simulink model "ammclib_mlib_vmac_s32k14x"  (Simulink 9.0)
settings: Solver=FixedStepDiscrete  StartTime=0.0  StopTime=5  FixedStep=0.001  RelTol=1e-3  EnableMultiTasking=on
InitFcn:
  | mbd_s32k_consistency_checks(bdroot(gcs));
undefined symbols (not defined in the file): LQFP
libraries: ammclib_bam_s32k14x x16, simulink x5, mbd_s32k1xx_ec_toolbox x2
Description:
  | This model tests the AMMCLIB MLIB VMAC blocks
  | 
  | Validation:
  | - Run the model in Simulation and compare the Inputs vs Outputs results.
  | - Open Freemaster (ammclib_mlib_vmac_s32k14x.pmp) and compare the HW results against the Simulated ones
settings Model: Creator=NXP MBDT Team  LastModifiedBy=nxf35172
settings DataIOCC: ExternalInput=off  InitialState=off  LimitDataPoints=on  SaveOutput=off  SignalLogging=off  SaveTime=off
settings OptimizationCC: DefaultParameterBehavior=Inlined  LifeSpan=1
settings DebuggingCC: SolverPrmCheckMsg=warning  InheritedTsInSrcMsg=none  SingleTaskRateTransMsg=error  ParameterPrecisionLossMsg=none  UnconnectedInputMsg=error  UnconnectedOutputMsg=error  UnconnectedLineMsg=error  AllowSymbolicDim=off  UnknownTsInhSupMsg=error  StateNameClashWarn=warning
settings HardwareCC: ProdLargestAtomicInteger=Long  ProdLargestAtomicFloat=Double  ProdEndianess=LittleEndian  ProdHWDeviceType=ARM Compatible->ARM Cortex
settings SFSimCC: MATLABDynamicMemAlloc=off
settings RTWCC: SystemTargetFile=mbd_s32k.tlc  MakeCommand=mbd_s32k_make_rtw COPY_MDLREF_INCLUDES=0  TemplateMakefile=mbd_s32k.tmf  Description=Model Based Design Toolbox S32K14x Code Generation Target
settings CodeAppCC: IgnoreCustomStorageClasses=off
settings STFCustomTargetCC: CombineOutputUpdateFcns=on  ERTCustomFileBanners=on  SupportContinuousTime=off  SupportNonInlinedSFcns=off  RemoveResetFunc=on  MATLABClassNameForMDSCustomization=Simulink.SoftwareTarget.ERTCustomization  GRTInterface=off  SystemTargetFile=mbd_s32k14.tlc
settings ERTTargetCC: MultiwordLength=2048  ParMdlRefBuildCompliant=off  CompOptLevelCompliant=off  ConcurrentExecutionCompliant=off  ModelStepFunctionPrototypeControlCompliant=off  CPPClassGenCompliant=off  UseToolchainInfoCompliant=off  InlinedParameterPlacement=NonHierarchical  ERTCustomFileTemplate=example_file_process.tlc  ConvertIfToSwitch=off  SuppressUnreachableDefaultCases=off

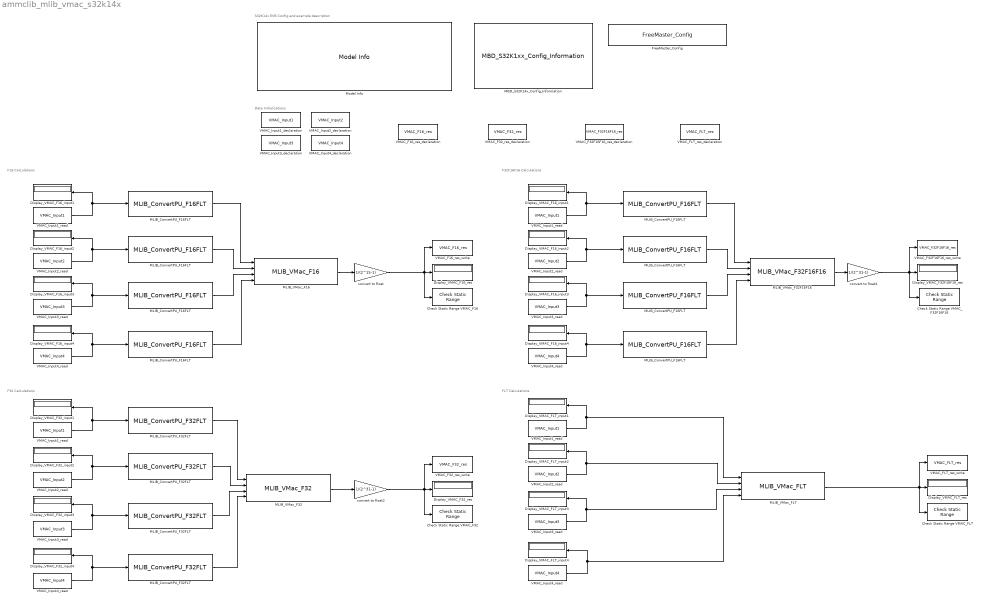
== system ammclib_mlib_vmac_s32k14x ==
  note: S32K14x EVB Config and example description
  note: Data Initializations
  note: F16 Calculations
  note: FLT Calculations
  note: F32F16F16 Calculations
  note: F32 Calculations
  "   MLIB_ConvertPU_F16FLT  " : ammclib_bam_s32k14x/MLIB/bam_f16/MLIB_ConvertPU_F16FLT
  "  MLIB_ConvertPU_F16FLT " : ammclib_bam_s32k14x/MLIB/bam_f16/MLIB_ConvertPU_F16FLT
  "  MLIB_ConvertPU_F16FLT   " : ammclib_bam_s32k14x/MLIB/bam_f16/MLIB_ConvertPU_F16FLT
  "  MLIB_ConvertPU_F16FLT     " : ammclib_bam_s32k14x/MLIB/bam_f16/MLIB_ConvertPU_F16FLT
  "  VMAC_Input4_read" : DataStoreRead  DataStoreName=VMAC_Input4
  " Display_VMAC_F16_input3" : Display
  " Display_VMAC_F16_input4" : Display
  " MLIB_ConvertPU_F16FLT" : ammclib_bam_s32k14x/MLIB/bam_f16/MLIB_ConvertPU_F16FLT
  " VMAC_Input3_read" : DataStoreRead  DataStoreName=VMAC_Input3
  Check Static Range VMAC_F16 : simulink/Model Verification/Check  Static Range  Description=0.194 <= u <= 0.196  max=0.196  max_included=on  min=0.194  min_included=on  enabled=on  stopWhenAssertionFail=on  export=off  icon=graphic
      settings: SourceProductName=Simulink  SourceProductBaseCode=SL
  "Check Static Range VMAC_F32 " : simulink/Model Verification/Check  Static Range  Description=0.194 <= u <= 0.196  max=0.196  max_included=on  min=0.194  min_included=on  enabled=on  stopWhenAssertionFail=on  export=off  icon=graphic
      settings: SourceProductName=Simulink  SourceProductBaseCode=SL
  "Check Static Range VMAC_F32F16F16 " : simulink/Model Verification/Check  Static Range  Description=0.194 <= u <= 0.196  max=0.196  max_included=on  min=0.194  min_included=on  enabled=on  stopWhenAssertionFail=on  export=off  icon=graphic
      settings: SourceProductName=Simulink  SourceProductBaseCode=SL
  "Check Static Range VMAC_FLT " : simulink/Model Verification/Check  Static Range  Description=0.194 <= u <= 0.196  max=0.196  max_included=on  min=0.194  min_included=on  enabled=on  stopWhenAssertionFail=on  export=off  icon=graphic
      settings: SourceProductName=Simulink  SourceProductBaseCode=SL
  Display_VMAC_F16_input{1..4} (4 alike) : Display
  "Display_VMAC_F16_input1   " : Display
  "Display_VMAC_F16_input2    " : Display
  Display_VMAC_F16_res : Display
  Display_VMAC_F32F16F16_res : Display
  Display_VMAC_F32_input1 : Display
  "Display_VMAC_F32_input2 " : Display
  Display_VMAC_F32_input3 : Display
  Display_VMAC_F32_input4 : Display
  Display_VMAC_F32_res : Display
  Display_VMAC_FLT_input{1..4} (4 alike) : Display
  Display_VMAC_FLT_res : Display
  FreeMaster_Config : mbd_s32k1xx_ec_toolbox/Utility Blocks/FreeMaster_Config  interface=LPUART1  baudrate=115200  rxd=PTC6: [LPUART1_RX | Receive]  txd=PTC7: [LPUART1_TX | Transmit]  mode=Short Interrupt  isr_prio=15  show_adv_opts=off  use_scope=on  max_scope_vars=8  use_recorder=on  max_rec_vars=8  rec_buff_size=1024  rec_timebase=0 milliseconds  comm_buffer_size_auto=on  comm_buffer_size=255  comm_rqueue_size_default=on  comm_rqueue_size=32
  MBD_S32K14x_Config_Information : mbd_s32k1xx_ec_toolbox/MBD_S32K1xx_Config_Information  Priority=0  mbdt_ver=0  disp_str=|  config_params=[]  mcu_target_name=S32K144  mcu_target_package=100-LQFP  mcu_target_sram_size=64KB  mcu_system_clock_freq=80  mcu_xtal_freq=External 8  mcu_steptick_timer=LPIT Channel 0  mcu_steptick_prio=15  ds_import_enable=on  target_compiler=GCC  target_memory=FLASH  gcc_target_compile_opts=-mcpu=cortex-m4 -mthumb -mfloat-abi=hard -mfpu=fpv4-sp-d16 -O1 -g -gstrict-dwarf  gcc_target_assemble_opts=-mcpu=cortex-m4 -mthumb -mfloat-abi=hard -mfpu=fpv4-sp-d16 -g  gcc_target_link_opts=-mcpu=cortex-m4 -mthumb -mfloat-abi=hard -mfpu=fpv4-sp-d16  gcc_target_default_lcf=on  gcc_target_user_lcf=S32K144_64_flash.ld  ghs_target_compile_opts=-cpu=cortexm4f -thumb -DARM_MATH_CM4 -fpu=vfpv4_d16 -fsingle -Ogeneral -Wundef -Wimplicit-int -Wshadow -Wtrigraphs --no_commons --gnu_asm -gnu99 -gdwarf-2 -G  ghs_target_assemble_opts=-cpu=cortexm4f -fpu=vfpv4_d16  ghs_target_link_opts=-cpu=cortexm4f -thumb -fpu=vfpv4_d16  ghs_target_default_lcf=off  ghs_target_user_lcf=S32K144_64_flash.ld  iar_target_compile_opts=--cpu=Cortex-M4F --thumb --fpu=VFPv4_sp -Ol -e --debug --dlib_config normal  iar_target_assemble_opts=--cpu Cortex-M4F --thumb --fpu VFPv4_sp  iar_target_link_opts=--no_exceptions --vfe --inline  iar_target_default_lcf=off  iar_target_user_lcf=S32K144_64_flash.icf  pil_download_enable=off  rbl_download_enable=on  rbl_start_delay=5000000  rbl_download_interface=OpenSDA  rbl_restart_request=off  rbl_com_port=Custom  rbl_com_port_custom=COM1  pil_download_rate=57600  pil_opensda_drive=Custom  pil_opensda_drive_custom=D  pil_uart_instance=1  pil_uart_rx=PTC6: [LPUART1_RX | Receive]  pil_uart_tx=PTC7: [LPUART1_TX | Transmit]  FTM_PWM_PcrCheckEnDis=on  FTM_Input_Edge_Inputs_PcrCheckEnDis=on  FTM_Dual_Edge_Inputs_PcrCheckEnDis=on  FTM_Quadrature_Inputs_PcrCheckEnDis=on  FTM_Hall_Sensor_Inputs_PcrCheckEnDis=on  LPTMR_PcrCheckEnDis=on  PIT_PcrCheckEnDis=on  RTC_PcrCheckEnDis=on  FlexCAN_PcrCheckEnDis=on  LIN_PcrCheckEnDis=on  FlexIO_PcrCheckEnDis=on  LPI2C_PcrCheckEnDis=on  LPSPI_PcrCheckEnDis=on  LPUART_PcrCheckEnDis=on  CMP_PcrCheckEnDis=on  GPIO_OutputPcrCheckEnDis=on  GPIO_InputPcrCheckEnDis=on  SBC_PcrCheckEnDis=on  AMMCLIB_PcrCheckEnDis=on  FM_PcrCheckEnDis=on  Profile_PcrCheckEnDis=on  ConfigParams_PcrCheckEnDis=on  ModelRef_PcrCheckEnDis=on  PDB0_PcrCheckEnDis=on  CSEc_PcrCheckEnDis=on  eDMA_PcrCheckEnDis=on  ADC_PcrCheckEnDis=on  WDOG_PcrCheckEnDis=on
      | Target : S32K142-16KB_SRAM
      | Package : 100-pin
      | System clock : 80 MHz
      | XTAL clock : External 8 MHz
      | Compiler : GCC
      | Target Type : FLASH
      | Download Code after build : (OpenSDA: E)
      | Step Tick Interrupt Priority : 15
  MLIB_ConvertPU_F16FLT : ammclib_bam_s32k14x/MLIB/bam_f16/MLIB_ConvertPU_F16FLT
  "MLIB_ConvertPU_F16FLT " : ammclib_bam_s32k14x/MLIB/bam_f16/MLIB_ConvertPU_F16FLT
  "MLIB_ConvertPU_F16FLT    " : ammclib_bam_s32k14x/MLIB/bam_f16/MLIB_ConvertPU_F16FLT
  MLIB_ConvertPU_F32FLT : ammclib_bam_s32k14x/MLIB/bam_f32/MLIB_ConvertPU_F32FLT
  "MLIB_ConvertPU_F32FLT " : ammclib_bam_s32k14x/MLIB/bam_f32/MLIB_ConvertPU_F32FLT
  "MLIB_ConvertPU_F32FLT   " : ammclib_bam_s32k14x/MLIB/bam_f32/MLIB_ConvertPU_F32FLT
  "MLIB_ConvertPU_F32FLT    " : ammclib_bam_s32k14x/MLIB/bam_f32/MLIB_ConvertPU_F32FLT
  MLIB_VMac_F16 : ammclib_bam_s32k14x/MLIB/bam_f16/MLIB_VMac_F16
  MLIB_VMac_F32 : ammclib_bam_s32k14x/MLIB/bam_f32/MLIB_VMac_F32
  MLIB_VMac_F32F16F16 : ammclib_bam_s32k14x/MLIB/bam_f32f16f16/MLIB_VMac_F32F16F16
  MLIB_VMac_FLT : ammclib_bam_s32k14x/MLIB/bam_flt/MLIB_VMac_FLT
  Model Info : simulink/Model-Wide Utilities/Model Info  Frame=off  DisplayStringWithTags=|  HorizontalTextAlignment=Left  LeftAlignmentValue=0.02
      | Model Name: %<ModelName>
      | 
      | Description: %<Description>
  VMAC_F16_res_declaration : DataStoreMemory  Priority=2  DataStoreName=VMAC_F16_res  ReadBeforeWriteMsg=warning  WriteAfterWriteMsg=warning  WriteAfterReadMsg=warning  ShowAdditionalParam=off  OutDataTypeStr=single
  VMAC_F16_res_write : DataStoreWrite  DataStoreName=VMAC_F16_res
  VMAC_F32F16F16_res_declaration : DataStoreMemory  Priority=2  DataStoreName=VMAC_F32F16F16_res  ReadBeforeWriteMsg=warning  WriteAfterWriteMsg=warning  WriteAfterReadMsg=warning  ShowAdditionalParam=off  OutDataTypeStr=single
  VMAC_F32F16F16_res_write : DataStoreWrite  DataStoreName=VMAC_F32F16F16_res
  VMAC_F32_res_declaration : DataStoreMemory  Priority=2  DataStoreName=VMAC_F32_res  ReadBeforeWriteMsg=warning  WriteAfterWriteMsg=warning  WriteAfterReadMsg=warning  ShowAdditionalParam=off  OutDataTypeStr=single
  VMAC_F32_res_write : DataStoreWrite  DataStoreName=VMAC_F32_res
  VMAC_FLT_res_declaration : DataStoreMemory  Priority=2  DataStoreName=VMAC_FLT_res  ReadBeforeWriteMsg=warning  WriteAfterWriteMsg=warning  WriteAfterReadMsg=warning  ShowAdditionalParam=off  OutDataTypeStr=single
  VMAC_FLT_res_write : DataStoreWrite  DataStoreName=VMAC_FLT_res
  VMAC_Input1_declaration : DataStoreMemory  Priority=1  DataStoreName=VMAC_Input1  WriteAfterWriteMsg=warning  WriteAfterReadMsg=warning  InitialValue=0.25  ShowAdditionalParam=off  OutMin=-1  OutMax=1  OutDataTypeStr=single
  VMAC_Input1_read : DataStoreRead  DataStoreName=VMAC_Input1
  "VMAC_Input1_read " : DataStoreRead  DataStoreName=VMAC_Input1
  "VMAC_Input1_read  " : DataStoreRead  DataStoreName=VMAC_Input1
  "VMAC_Input1_read   " : DataStoreRead  DataStoreName=VMAC_Input1
  VMAC_Input2_declaration : DataStoreMemory  Priority=1  DataStoreName=VMAC_Input2  WriteAfterWriteMsg=warning  WriteAfterReadMsg=warning  InitialValue=0.15  ShowAdditionalParam=off  OutMin=-1  OutMax=1  OutDataTypeStr=single
  VMAC_Input2_read : DataStoreRead  DataStoreName=VMAC_Input2
  "VMAC_Input2_read " : DataStoreRead  DataStoreName=VMAC_Input2
  "VMAC_Input2_read   " : DataStoreRead  DataStoreName=VMAC_Input2
  "VMAC_Input2_read     " : DataStoreRead  DataStoreName=VMAC_Input2
  VMAC_Input3_declaration : DataStoreMemory  Priority=1  DataStoreName=VMAC_Input3  WriteAfterWriteMsg=warning  WriteAfterReadMsg=warning  InitialValue=0.35  ShowAdditionalParam=off  OutMin=-1  OutMax=1  OutDataTypeStr=single
  VMAC_Input3_read : DataStoreRead  DataStoreName=VMAC_Input3
  "VMAC_Input3_read   " : DataStoreRead  DataStoreName=VMAC_Input3
  "VMAC_Input3_read    " : DataStoreRead  DataStoreName=VMAC_Input3
  VMAC_Input4_declaration : DataStoreMemory  Priority=1  DataStoreName=VMAC_Input4  WriteAfterWriteMsg=warning  WriteAfterReadMsg=warning  InitialValue=0.45  ShowAdditionalParam=off  OutMin=-1  OutMax=1  OutDataTypeStr=single
  VMAC_Input4_read : DataStoreRead  DataStoreName=VMAC_Input4
  "VMAC_Input4_read  " : DataStoreRead  DataStoreName=VMAC_Input4
  "VMAC_Input4_read     " : DataStoreRead  DataStoreName=VMAC_Input4
  convert to float : Gain  Gain=1/(2^15-1)  OutDataTypeStr=Inherit: Inherit via back propagation
  convert to float2 : Gain  Gain=1/(2^31-1)  OutDataTypeStr=Inherit: Inherit via back propagation
  convert to float4 : Gain  Gain=1/(2^31-1)  OutDataTypeStr=Inherit: Inherit via back propagation
  wires:
  VMAC_Input1_read/1 -> Display_VMAC_F16_input1/1, MLIB_ConvertPU_F16FLT/1
  convert to float/1 -> VMAC_F16_res_write/1, Display_VMAC_F16_res/1, Check Static Range VMAC_F16/1
  MLIB_VMac_F16/1 -> convert to float/1
  VMAC_Input2_read/1 -> Display_VMAC_F16_input2/1, "MLIB_ConvertPU_F16FLT "/1
  MLIB_ConvertPU_F16FLT/1 -> MLIB_VMac_F16/1
  "MLIB_ConvertPU_F16FLT "/1 -> MLIB_VMac_F16/2
  "VMAC_Input1_read "/1 -> MLIB_ConvertPU_F32FLT/1, Display_VMAC_F32_input1/1
  convert to float2/1 -> "Check Static Range VMAC_F32 "/1, VMAC_F32_res_write/1, Display_VMAC_F32_res/1
  MLIB_VMac_F32/1 -> convert to float2/1
  "VMAC_Input2_read "/1 -> "Display_VMAC_F32_input2 "/1, "MLIB_ConvertPU_F32FLT "/1
  MLIB_ConvertPU_F32FLT/1 -> MLIB_VMac_F32/1
  "MLIB_ConvertPU_F32FLT "/1 -> MLIB_VMac_F32/2
  MLIB_VMac_FLT/1 -> "Check Static Range VMAC_FLT "/1, VMAC_FLT_res_write/1, Display_VMAC_FLT_res/1
  "VMAC_Input1_read  "/1 -> MLIB_VMac_FLT/1, Display_VMAC_FLT_input1/1
  "VMAC_Input2_read   "/1 -> Display_VMAC_FLT_input2/1, MLIB_VMac_FLT/2
  convert to float4/1 -> "Check Static Range VMAC_F32F16F16 "/1, VMAC_F32F16F16_res_write/1, Display_VMAC_F32F16F16_res/1
  MLIB_VMac_F32F16F16/1 -> convert to float4/1
  VMAC_Input3_read/1 -> "MLIB_ConvertPU_F16FLT    "/1, Display_VMAC_F16_input3/1
  VMAC_Input4_read/1 -> Display_VMAC_F16_input4/1, " MLIB_ConvertPU_F16FLT"/1
  "MLIB_ConvertPU_F16FLT    "/1 -> MLIB_VMac_F16/3
  " MLIB_ConvertPU_F16FLT"/1 -> MLIB_VMac_F16/4
  "VMAC_Input3_read   "/1 -> "MLIB_ConvertPU_F32FLT   "/1, Display_VMAC_F32_input3/1
  "VMAC_Input4_read  "/1 -> Display_VMAC_F32_input4/1, "MLIB_ConvertPU_F32FLT    "/1
  "MLIB_ConvertPU_F32FLT   "/1 -> MLIB_VMac_F32/3
  "MLIB_ConvertPU_F32FLT    "/1 -> MLIB_VMac_F32/4
  "VMAC_Input1_read   "/1 -> "Display_VMAC_F16_input1   "/1, "  MLIB_ConvertPU_F16FLT "/1
  "VMAC_Input2_read     "/1 -> "Display_VMAC_F16_input2    "/1, "  MLIB_ConvertPU_F16FLT   "/1
  "  MLIB_ConvertPU_F16FLT "/1 -> MLIB_VMac_F32F16F16/1
  "  MLIB_ConvertPU_F16FLT   "/1 -> MLIB_VMac_F32F16F16/2
  " VMAC_Input3_read"/1 -> "  MLIB_ConvertPU_F16FLT     "/1, " Display_VMAC_F16_input3"/1
  "  VMAC_Input4_read"/1 -> " Display_VMAC_F16_input4"/1, "   MLIB_ConvertPU_F16FLT  "/1
  "  MLIB_ConvertPU_F16FLT     "/1 -> MLIB_VMac_F32F16F16/3
  "   MLIB_ConvertPU_F16FLT  "/1 -> MLIB_VMac_F32F16F16/4
  "VMAC_Input3_read    "/1 -> Display_VMAC_FLT_input3/1, MLIB_VMac_FLT/3
  "VMAC_Input4_read     "/1 -> Display_VMAC_FLT_input4/1, MLIB_VMac_FLT/4
